simulink library "casper_library"  (Simulink 6.2)
PostLoadFcn:
  | % Stub definitions for mask variables
  | delay_depth=16;
  | n_bits=8;
  | bin_pt=7;
values from neighbouring files (symbols this model uses):
  add_latency = get_var('add_latency', 'defaults', defaults, varargin{:})    [biplex_core_init.m]    (also in butterfly_direct_init.m; dec_fir_init.m = get_var('add_latency','defaults', defaults, varargin{:}); fft_biplex_real_4x_init.m; fft_direct_init.m)
  BitWidth = get_var('BitWidth', 'defaults', defaults, varargin{:})    [biplex_core_init.m]    (also in butterfly_direct_init.m; fft_biplex_init.m; fft_biplex_real_2x_init.m; fft_biplex_real_4x_init.m)
  blockCountBits = ceil(log2(numBlocks))    [address_gen_vacc_v2_mask.m]
  blockRowBits = 0    [address_gen_vacc_v2_mask.m]
  mult_latency = get_var('mult_latency', 'defaults', defaults, varargin{:})    [biplex_core_init.m]    (also in butterfly_direct_init.m; dec_fir_init.m = get_var('mult_latency','defaults', defaults, varargin{:}); fft_biplex_real_4x_init.m; fft_direct_init.m)
  n_inputs = get_var('n_inputs', 'defaults', defaults, varargin{:})    [adder_tree_init.m]    (also in barrel_switcher_init.m; dec_fir_init.m = get_var('n_inputs','defaults', defaults, varargin{:}); fft_init.m; fft_unscrambler_init.m)
undefined symbols (not defined in the file or in its folder): acc_len, ant_bits, bit_growth, bit_rev, BitWidthIn, cmult_4bit_br, cmult_4bit_em, cmult_4bit_sl, CoeffBitWidth, DelayLen, n_ants, n_bits_out, pfb_coeff_gen_calc, PFBSize
libraries: xbsIndex_r3 x2630, casper_library x215, xps_library x24, fft_library x4
(part 4 of 21)

== system casper_library/Downconverter/fir_dbl_col ==
  real1 : Inport  Port=1  LatchInput=off
  imag1 : Inport  Port=2  LatchInput=off
  real2 : Inport  Port=3  LatchInput=off
  imag2 : Inport  Port=4  LatchInput=off
  real_back1 : Inport  Port=5  LatchInput=off
  imag_back1 : Inport  Port=6  LatchInput=off
  real_back2 : Inport  Port=7  LatchInput=off
  imag_back2 : Inport  Port=8  LatchInput=off
  adder_tree1 : Subsystem  AncestorBlock=casper_library/Misc/adder_tree  mask(adder_tree){n_inputs=2, latency=2}
      mask prompts: n_inputs "Number of Inputs"; latency "Add Latency"
      mask help: Sums all inputs using a tree of adds and delays.
      mask init:
      | adder_tree_init(gcb, ...
      |     'n_inputs', n_inputs, ...
      |     'latency', latency);
      settings: AttributesFormatString=latency 2
      mask Help: eval('xlWeb([getenv(''MLIB_ROOT''), ''\doc\html\sp_adder_tree\sp_adder_tree.html''])')
  adder_tree2 : Subsystem  AncestorBlock=casper_library/Misc/adder_tree  mask(adder_tree){n_inputs=2, latency=2}
      mask prompts: n_inputs "Number of Inputs"; latency "Add Latency"
      mask help: Sums all inputs using a tree of adds and delays.
      mask init:
      | adder_tree_init(gcb, ...
      |     'n_inputs', n_inputs, ...
      |     'latency', latency);
      settings: AttributesFormatString=latency 2
      mask Help: eval('xlWeb([getenv(''MLIB_ROOT''), ''\doc\html\sp_adder_tree\sp_adder_tree.html''])')
  c1 : xbsIndex_r3/Constant  const=1  equ=P=C  arith_type=Unsigned  n_bits=1  bin_pt=0  opselect=C  inp2=PCIN>>17  opr=+  inp1=P  carry=CIN  iostate=0  explicit_period=on  period=1  dbl_ovrd=off
  c2 : xbsIndex_r3/Constant  const=1  equ=P=C  arith_type=Unsigned  n_bits=1  bin_pt=0  opselect=C  inp2=PCIN>>17  opr=+  inp1=P  carry=CIN  iostate=0  explicit_period=on  period=1  dbl_ovrd=off
  fir_dbl_tap1 : Subsystem  AncestorBlock=casper_library/Downconverter/fir_dbl_tap  mask(fir_dbl_tap){factor=0.1, add_latency=2, mult_latency=3}
      mask prompts: add_latency "Add latency"; mult_latency "Mult latency"
  fir_dbl_tap2 : Subsystem  AncestorBlock=casper_library/Downconverter/fir_dbl_tap  mask(fir_dbl_tap){factor=0.2, add_latency=2, mult_latency=3}
      mask prompts: add_latency "Add latency"; mult_latency "Mult latency"
  real_out1 : Outport
  imag_out1 : Outport  Port=2
  real_out2 : Outport  Port=3
  imag_out2 : Outport  Port=4
  real_back_out1 : Outport  Port=5
  imag_back_out1 : Outport  Port=6
  real_back_out2 : Outport  Port=7
  imag_back_out2 : Outport  Port=8
  real_sum : Outport  Port=9
  imag_sum : Outport  Port=10
  wires:
  c1/1 -> adder_tree1/1(sync)
  c2/1 -> adder_tree2/1(sync)
  adder_tree1/2(dout) -> real_sum/1
  adder_tree2/2(dout) -> imag_sum/1
  real1/1 -> fir_dbl_tap1/1(a)
  imag1/1 -> fir_dbl_tap1/2(b)
  real_back2/1 -> fir_dbl_tap1/3(c)
  imag_back2/1 -> fir_dbl_tap1/4(d)
  fir_dbl_tap1/1(a_out) -> real_out1/1
  fir_dbl_tap1/2(b_out) -> imag_out1/1
  fir_dbl_tap1/3(c_out) -> real_back_out2/1
  fir_dbl_tap1/4(d_out) -> imag_back_out2/1
  fir_dbl_tap1/5(real) -> adder_tree1/2(din1)
  fir_dbl_tap1/6(imag) -> adder_tree2/2(din1)
  real2/1 -> fir_dbl_tap2/1(a)
  imag2/1 -> fir_dbl_tap2/2(b)
  real_back1/1 -> fir_dbl_tap2/3(c)
  imag_back1/1 -> fir_dbl_tap2/4(d)
  fir_dbl_tap2/1(a_out) -> real_out2/1
  fir_dbl_tap2/2(b_out) -> imag_out2/1
  fir_dbl_tap2/3(c_out) -> real_back_out1/1
  fir_dbl_tap2/4(d_out) -> imag_back_out1/1
  fir_dbl_tap2/5(real) -> adder_tree1/3(din2)
  fir_dbl_tap2/6(imag) -> adder_tree2/3(din2)

== system casper_library/Downconverter/fir_dbl_tap ==
  a : Inport  Port=1  LatchInput=off
  b : Inport  Port=2  LatchInput=off
  c : Inport  Port=3  LatchInput=off
  d : Inport  Port=4  LatchInput=off
  AddSub : xbsIndex_r3/AddSub  mode=Addition  precision=User Defined  arith_type="Signed  (2's comp)"  n_bits=18  bin_pt=16  quantization=Truncate  overflow=Wrap  latency=add_latency  explicit_period=on  period=1  use_carryin=off  use_carryout=off  en=off  dbl_ovrd=off  show_param=off  use_core=on  pipeline=off  use_rpm=on  gen_core=off
      settings: xl_area=[0, 0, 0, 0, 0, 0, 0]
  AddSub1 : xbsIndex_r3/AddSub  mode=Addition  precision=User Defined  arith_type="Signed  (2's comp)"  n_bits=18  bin_pt=16  quantization=Truncate  overflow=Wrap  latency=add_latency  explicit_period=on  period=1  use_carryin=off  use_carryout=off  en=off  dbl_ovrd=off  show_param=off  use_core=on  pipeline=off  use_rpm=on  gen_core=off
      settings: xl_area=[0, 0, 0, 0, 0, 0, 0]
  Constant : xbsIndex_r3/Constant  const=factor  equ=P=C  arith_type="Signed  (2's comp)"  n_bits=18  bin_pt=17  opselect=C  inp2=PCIN>>17  opr=+  inp1=P  carry=CIN  iostate=0  explicit_period=on  period=1  dbl_ovrd=off
  Mult : xbsIndex_r3/Mult  precision=Full  arith_type="Signed  (2's comp)"  n_bits=18  bin_pt=17  quantization=Truncate  overflow=Wrap  latency=mult_latency  explicit_period=off  period=1  en=off  dbl_ovrd=off  show_param=on  mult_type=Parallel  oversample=2  use_embedded=on  pipeline=on  use_rpm=off  placement_style=Rectangular Shape  gen_core=off
      settings: xl_area=[0, 0, 0, 0, 0, 0, 0]
  Mult1 : xbsIndex_r3/Mult  precision=Full  arith_type="Signed  (2's comp)"  n_bits=18  bin_pt=17  quantization=Truncate  overflow=Wrap  latency=mult_latency  explicit_period=off  period=1  en=off  dbl_ovrd=off  show_param=on  mult_type=Parallel  oversample=2  use_embedded=on  pipeline=on  use_rpm=off  placement_style=Rectangular Shape  gen_core=off
      settings: xl_area=[0, 0, 0, 0, 0, 0, 0]
  Register{,1..3} (4 alike) : xbsIndex_r3/Register  init=0  reg_only_valid=off  explicit_period=on  period=1  rst=off  en=off  out_en=off  dbl_ovrd=off  show_param=off
      settings: xl_area=[0, 0, 0, 0, 0, 0, 0]
  a_out : Outport
  b_out : Outport  Port=2
  c_out : Outport  Port=3
  d_out : Outport  Port=4
  real : Outport  Port=5
  imag : Outport  Port=6
  wires:
  AddSub1/1 -> Mult/2
  AddSub/1 -> Mult1/2
  d/1 -> AddSub1/2, Register3/1
  c/1 -> AddSub/2, Register2/1
  b/1 -> AddSub1/1, Register1/1
  a/1 -> AddSub/1, Register/1
  Register2/1 -> c_out/1
  Register3/1 -> d_out/1
  Mult1/1 -> real/1
  Mult/1 -> imag/1
  Constant/1 -> Mult1/1, Mult/1
  Register/1 -> a_out/1
  Register1/1 -> b_out/1

== system casper_library/Downconverter/fir_tap ==
  a : Inport  Port=1  LatchInput=off
  b : Inport  Port=2  LatchInput=off
  Constant : xbsIndex_r3/Constant  const=factor  equ=P=C  arith_type="Signed  (2's comp)"  n_bits=18  bin_pt=17  opselect=C  inp2=PCIN>>17  opr=+  inp1=P  carry=CIN  iostate=0  explicit_period=on  period=1  dbl_ovrd=off
  Mult : xbsIndex_r3/Mult  precision=Full  arith_type="Signed  (2's comp)"  n_bits=18  bin_pt=17  quantization=Truncate  overflow=Wrap  latency=latency  explicit_period=on  period=1  en=off  dbl_ovrd=off  show_param=on  mult_type=Parallel  oversample=2  use_embedded=on  pipeline=on  use_rpm=off  placement_style=Rectangular Shape  gen_core=off
      settings: xl_area=[0, 0, 0, 0, 0, 0, 0]
  Mult1 : xbsIndex_r3/Mult  precision=Full  arith_type="Signed  (2's comp)"  n_bits=18  bin_pt=17  quantization=Truncate  overflow=Wrap  latency=latency  explicit_period=on  period=1  en=off  dbl_ovrd=off  show_param=on  mult_type=Parallel  oversample=2  use_embedded=on  pipeline=on  use_rpm=off  placement_style=Rectangular Shape  gen_core=off
      settings: xl_area=[0, 0, 0, 0, 0, 0, 0]
  Register : xbsIndex_r3/Register  init=0  reg_only_valid=off  explicit_period=on  period=1  rst=off  en=off  out_en=off  dbl_ovrd=off  show_param=off
      settings: xl_area=[0, 0, 0, 0, 0, 0, 0]
  Register1 : xbsIndex_r3/Register  init=0  reg_only_valid=off  explicit_period=on  period=1  rst=off  en=off  out_en=off  dbl_ovrd=off  show_param=off
      settings: xl_area=[0, 0, 0, 0, 0, 0, 0]
  a_out : Outport
  b_out : Outport  Port=2
  real : Outport  Port=3
  imag : Outport  Port=4
  wires:
  Register1/1 -> b_out/1
  Register/1 -> a_out/1
  Constant/1 -> Mult/1, Mult1/1
  a/1 -> Register/1, Mult1/2
  Mult/1 -> imag/1
  b/1 -> Register1/1, Mult/2
  Mult1/1 -> real/1

== system casper_library/Downconverter/lo_const ==
  const : xbsIndex_r3/Constant  const=real(exp(phase*1j))  equ=P=C  arith_type="Signed  (2's comp)"  n_bits=n_bits  bin_pt=n_bits - 1  opselect=C  inp2=PCIN>>17  opr=+  inp1=P  carry=CIN  iostate=0  explicit_period=on  period=1  dbl_ovrd=off
  const1 : xbsIndex_r3/Constant  const=-imag(exp(phase*1j))  equ=P=C  arith_type="Signed  (2's comp)"  n_bits=n_bits  bin_pt=n_bits - 1  opselect=C  inp2=PCIN>>17  opr=+  inp1=P  carry=CIN  iostate=0  explicit_period=on  period=1  dbl_ovrd=off
  sin : Outport
  cos : Outport  Port=2
  wires:
  const/1 -> cos/1
  const1/1 -> sin/1

== system casper_library/Downconverter/lo_osc ==
  sync : Inport  Port=1  LatchInput=off
  SineCosine : xbsIndex_r3/SineCosine  mode=Sine and Cosine  neg_sin=on  neg_cos=off  n_bits=n_bits  latency=latency  sym_output=off  explicit_period=off  period=1  en=off  dbl_ovrd=off  show_param=off  mem_type=Block RAM  pipeline=on  use_rpm=on  gen_core=off
      settings: xl_area=[0, 0, 0, 0, 0, 0, 0]
  counter : xbsIndex_r3/Counter  cnt_type=Free Running  n_bits=counter_width  bin_pt=0  arith_type=Unsigned  start_count=counter_start  cnt_to=Inf  cnt_by_val=counter_step  operation=Up  explicit_period=off  period=1  load_pin=off  rst=on  en=off  dbl_ovrd=off  show_param=off  use_rpm=on  gen_core=off
      settings: xl_area=[0, 0, 0, 0, 0, 0, 0]
  sin : Outport
  cos : Outport  Port=2
  wires:
  counter/1 -> SineCosine/1
  SineCosine/2 -> cos/1
  SineCosine/1 -> sin/1
  sync/1 -> counter/1

== system casper_library/Downconverter/mixer ==
  sync : Inport  Port=1  LatchInput=off
  din1 : Inport  Port=2  LatchInput=off
  din2 : Inport  Port=3  LatchInput=off
  din3 : Inport  Port=4  LatchInput=off
  din4 : Inport  Port=5  LatchInput=off
  dds : Subsystem  AncestorBlock=casper_library/Downconverter/dds  mask(dds){freq_div=16, freq=1, num_lo=4, n_bits=8, latency=2}
      mask prompts: freq_div "Frequency divisions (M)"; freq "Frequency (? / M*2pi)"; num_lo "Parallel LOs"; n_bits "Bit Width"
      mask init:
      | dds_init(gcb, ...
      |     'freq_div', freq_div, ...
      |     'freq', freq, ...
      |     'num_lo', num_lo, ...
      |     'n_bits', n_bits, ...
      |     'latency', latency);
      settings: AttributesFormatString=lo at -1/16
  delay : xbsIndex_r3/Delay  latency=3  reg_retiming=off  explicit_period=off  period=1  en=off  accept_only_valid=off  init_zero=on  dbl_ovrd=off  show_param=off
      settings: xl_area=[0, 0, 0, 0, 0, 0, 0]
  rcmult1 : Subsystem  AncestorBlock=casper_library/Downconverter/rcmult  mask(rcmult){latency=3}
  rcmult2 : Subsystem  AncestorBlock=casper_library/Downconverter/rcmult  mask(rcmult){latency=3}
  rcmult3 : Subsystem  AncestorBlock=casper_library/Downconverter/rcmult  mask(rcmult){latency=3}
  rcmult4 : Subsystem  AncestorBlock=casper_library/Downconverter/rcmult  mask(rcmult){latency=3}
  sync_out : Outport
  real1 : Outport  Port=2
  imag1 : Outport  Port=3
  real2 : Outport  Port=4
  imag2 : Outport  Port=5
  real3 : Outport  Port=6
  imag3 : Outport  Port=7
  real4 : Outport  Port=8
  imag4 : Outport  Port=9
  wires:
  sync/1 -> delay/1
  delay/1 -> sync_out/1
  din1/1 -> rcmult1/1(d)
  dds/1(sin0) -> rcmult1/2(sin)
  dds/2(cos0) -> rcmult1/3(cos)
  rcmult1/1(real) -> real1/1
  rcmult1/2(imag) -> imag1/1
  din2/1 -> rcmult2/1(d)
  dds/3(sin1) -> rcmult2/2(sin)
  dds/4(cos1) -> rcmult2/3(cos)
  rcmult2/1(real) -> real2/1
  rcmult2/2(imag) -> imag2/1
  din3/1 -> rcmult3/1(d)
  dds/5(sin2) -> rcmult3/2(sin)
  dds/6(cos2) -> rcmult3/3(cos)
  rcmult3/1(real) -> real3/1
  rcmult3/2(imag) -> imag3/1
  din4/1 -> rcmult4/1(d)
  dds/7(sin3) -> rcmult4/2(sin)
  dds/8(cos3) -> rcmult4/3(cos)
  rcmult4/1(real) -> real4/1
  rcmult4/2(imag) -> imag4/1

== system casper_library/Downconverter/rcmult ==
  d : Inport  Port=1  LatchInput=off
  sin : Inport  Port=2  LatchInput=off
  cos : Inport  Port=3  LatchInput=off
  Mult : xbsIndex_r3/Mult  precision=Full  arith_type="Signed  (2's comp)"  n_bits=BitWidth  bin_pt=BitWidth-1  quantization=Truncate  overflow=Wrap  latency=latency  explicit_period=off  period=1  en=off  dbl_ovrd=off  show_param=on  mult_type=Parallel  oversample=2  use_embedded=on  pipeline=on  use_rpm=off  placement_style=Rectangular Shape  gen_core=off
      settings: xl_area=[0, 0, 0, 0, 0, 0, 0]
  Mult1 : xbsIndex_r3/Mult  precision=Full  arith_type="Signed  (2's comp)"  n_bits=BitWidth  bin_pt=BitWidth-1  quantization=Truncate  overflow=Wrap  latency=latency  explicit_period=off  period=1  en=off  dbl_ovrd=off  show_param=on  mult_type=Parallel  oversample=2  use_embedded=on  pipeline=on  use_rpm=off  placement_style=Rectangular Shape  gen_core=off
      settings: xl_area=[0, 0, 0, 0, 0, 0, 0]
  real : Outport
  imag : Outport  Port=2
  wires:
  Mult1/1 -> imag/1
  Mult/1 -> real/1
  d/1 -> Mult1/1, Mult/1
  sin/1 -> Mult1/2
  cos/1 -> Mult/2

== system casper_library/FFTs/Twiddle ==
  coeff_gen : Subsystem
  twiddle : Subsystem  BlockChoice=twiddle_coeff_0
      settings: TemplateBlock=self  MemberBlocks=twiddle_coeff_0,twiddle_coeff_1,twiddle_general_3mult,twiddle_general_4mult,twiddle_stage_2
  twiddle_coeff_0 : Subsystem  mask{BitWidth=18, add_latency=3, mult_latency=4, bram_latency=4}
      mask prompts: BitWidth "Bit Width"; add_latency "Add Latency"; mult_latency "Mult Latency"; bram_latency "BRAM Latency"
      mask init:
      | disp(gcb);
  twiddle_coeff_1 : Subsystem  mask{BitWidth=18, add_latency=3, mult_latency=4, bram_latency=4}
      mask prompts: BitWidth "Bit Width"; add_latency "Add Latency"; mult_latency "Mult Latency"; bram_latency "BRAM Latency"
  twiddle_general_3mult : Subsystem  mask{Coeffs=[0], StepPeriod=0, BitWidth=18, add_latency=3, mult_latency=4, bram_latency=4}
      mask prompts: Coeffs "Coefficients:"; StepPeriod "Coefficient Step Period (2^?)"; BitWidth "Bit Width"; add_latency "Add Latency"; mult_latency "Mult Latency"; bram_latency "BRAM Latency"
  twiddle_general_4mult : Subsystem  mask{Coeffs=[0], StepPeriod=0, BitWidth=18, add_latency=3, mult_latency=4, bram_latency=4}
      mask prompts: Coeffs "Coefficients:"; StepPeriod "Coefficient Step Period (2^?)"; BitWidth "Bit Width"; add_latency "Add Latency"; mult_latency "Mult Latency"; bram_latency "BRAM Latency"
  twiddle_stage_2 : Subsystem  mask{FFTSize=5, BitWidth=18, add_latency=3, mult_latency=4, bram_latency=4}
      mask prompts: FFTSize "Size of FFT: (2^?)"; BitWidth "Bit Width"; add_latency "Add Latency"; mult_latency "Mult Latency"; bram_latency "BRAM Latency"

== system casper_library/FFTs/biplex_core ==
  pol1 : Inport  Port=1  LatchInput=off
  pol2 : Inport  Port=2  LatchInput=off
  sync : Inport  Port=3  LatchInput=off
  shift : Inport  Port=4  LatchInput=off
  fft_stage_1 : Subsystem  mask(fft_stage_n){FFTSize=3, FFTStage=1, BitWidth=18, use_bram=0, CoeffBram=0, MaxCoeffNum=16, quantization=Truncate, overflow=Wrap, add_latency=2, mult_latency=3, bram_latency=2}
      mask prompts: FFTSize "Size of FFT: (2^? pnts)"; FFTStage "Stage of FFT:"; BitWidth "Output Bitwidth:"; use_bram "Implement Delays in BRAM:"; CoeffBram "Store Coefficients in BRAM:"; MaxCoeffNum "Maximum Coefficient Depth: (2^?)"; quantization "Quantization Behavior"; overflow "Overflow Behavior"; add_latency "Add Latency"; mult_latency "Mult Latency"; bram_latency "BRAM Latency"
      mask init: same as casper_library/FFTs/fft_stage_n
      settings: AttributesFormatString=FFTSize=3, FFTStage=1, BitWidth=18
      mask StyleString: edit,edit,edit,edit,edit,edit,popup(Truncate|Round  (unbiased: +/- Inf)|Round  (unbiased: Even Values)),popup(Wrap|Saturate|Error),edit,edit,edit
  fft_stage_2 : casper_library/FFTs/fft_stage_n  FFTSize=3  FFTStage=2  BitWidth=18  use_bram=0  CoeffBram=0  MaxCoeffNum=16  quantization=Truncate  overflow=Wrap  add_latency=2  mult_latency=3  bram_latency=2
      settings: AttributesFormatString=FFTSize=3, FFTStage=2, BitWidth=18
  fft_stage_3 : casper_library/FFTs/fft_stage_n  FFTSize=3  FFTStage=3  BitWidth=18  use_bram=0  CoeffBram=0  MaxCoeffNum=16  quantization=Truncate  overflow=Wrap  add_latency=2  mult_latency=3  bram_latency=2
      settings: AttributesFormatString=FFTSize=3, FFTStage=3, BitWidth=18
  out1 : Outport
  out2 : Outport  Port=2
  of : Outport  Port=3
  sync_out : Outport  Port=4
  wires:
  fft_stage_1/1(out1) -> fft_stage_2/1
  fft_stage_1/2(out2) -> fft_stage_2/2
  fft_stage_1/3(of) -> fft_stage_2/3
  fft_stage_1/4(sync_out) -> fft_stage_2/4
  shift/1 -> fft_stage_2/5, fft_stage_3/5, fft_stage_1/4(shift)
  fft_stage_2/1 -> fft_stage_3/1
  fft_stage_2/2 -> fft_stage_3/2
  fft_stage_2/3 -> fft_stage_3/3
  fft_stage_2/4 -> fft_stage_3/4
  pol1/1 -> fft_stage_1/1(in1)
  pol2/1 -> fft_stage_1/2(in2)
  sync/1 -> fft_stage_1/3(sync)
  fft_stage_3/1 -> out1/1
  fft_stage_3/2 -> out2/1
  fft_stage_3/3 -> of/1
  fft_stage_3/4 -> sync_out/1

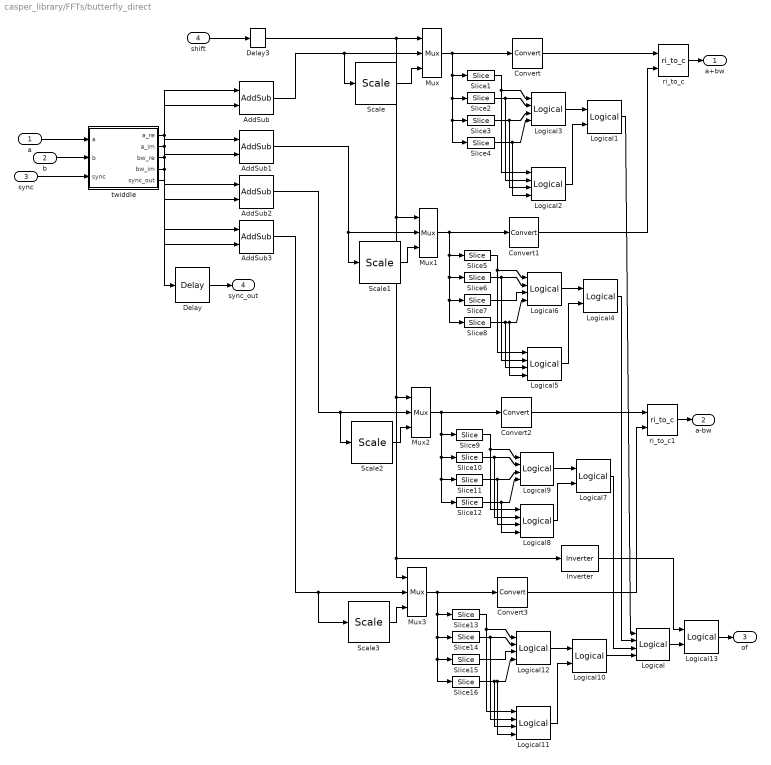
== system casper_library/FFTs/butterfly_direct ==
  a : Inport  Port=1  LatchInput=off
  b : Inport  Port=2  LatchInput=off
  sync : Inport  Port=3  LatchInput=off
  shift : Inport  Port=4  LatchInput=off
  AddSub : xbsIndex_r3/AddSub  mode=Addition  precision=Full  arith_type=Unsigned  n_bits=8  bin_pt=2  quantization=Truncate  overflow=Wrap  latency=add_latency  explicit_period=off  period=1  use_carryin=off  use_carryout=off  en=off  dbl_ovrd=off  show_param=on  use_core=on  pipeline=on  use_rpm=on  gen_core=on
      settings: xl_area=[0, 0, 0, 0, 0, 0, 0]
  AddSub1 : xbsIndex_r3/AddSub  mode=Addition  precision=Full  arith_type=Unsigned  n_bits=8  bin_pt=2  quantization=Truncate  overflow=Wrap  latency=add_latency  explicit_period=off  period=1  use_carryin=off  use_carryout=off  en=off  dbl_ovrd=off  show_param=on  use_core=on  pipeline=on  use_rpm=on  gen_core=on
      settings: xl_area=[0, 0, 0, 0, 0, 0, 0]
  AddSub2 : xbsIndex_r3/AddSub  mode=Subtraction  precision=Full  arith_type=Unsigned  n_bits=8  bin_pt=2  quantization=Truncate  overflow=Wrap  latency=add_latency  explicit_period=off  period=1  use_carryin=off  use_carryout=off  en=off  dbl_ovrd=off  show_param=on  use_core=on  pipeline=on  use_rpm=on  gen_core=on
      settings: xl_area=[0, 0, 0, 0, 0, 0, 0]
  AddSub3 : xbsIndex_r3/AddSub  mode=Subtraction  precision=Full  arith_type=Unsigned  n_bits=8  bin_pt=2  quantization=Truncate  overflow=Wrap  latency=add_latency  explicit_period=off  period=1  use_carryin=off  use_carryout=off  en=off  dbl_ovrd=off  show_param=on  use_core=on  pipeline=on  use_rpm=on  gen_core=on
      settings: xl_area=[0, 0, 0, 0, 0, 0, 0]
  Convert{,1..3} (4 alike) : xbsIndex_r3/Convert  arith_type="Signed  (2's comp)"  n_bits=BitWidth  bin_pt=BitWidth-1  quantization=Truncate  overflow=Wrap  latency=add_latency  explicit_period=off  period=1  dbl_ovrd=off  show_param=off  inserted_by_tool=off  pipeline=off
      settings: xl_area=[0, 0, 0, 0, 0, 0, 0]
  Delay : xbsIndex_r3/Delay  latency=2 * add_latency + 1  reg_retiming=off  explicit_period=off  period=1  en=off  accept_only_valid=off  init_zero=on  dbl_ovrd=off  show_param=off
      settings: xl_area=[0, 0, 0, 0, 0, 0, 0]
  Delay3 : xbsIndex_r3/Delay  latency=1  reg_retiming=off  explicit_period=off  period=1  en=off  accept_only_valid=off  init_zero=on  dbl_ovrd=off  show_param=off
      settings: xl_area=[0, 0, 0, 0, 0, 0, 0]
  Inverter : xbsIndex_r3/Inverter  latency=0  explicit_period=off  period=1  en=off  dbl_ovrd=off  show_param=off
      settings: xl_area=[0, 0, 0, 0, 0, 0, 0]
  Logical : xbsIndex_r3/Logical  logical_function=OR  inputs=4  precision=Full  arith_type=Unsigned  n_bits=8  bin_pt=2  align_bp=on  latency=1  explicit_period=off  period=1  en=off  dbl_ovrd=off  show_param=off
      settings: xl_area=[0, 0, 0, 0, 0, 0, 0]
  Logical{1,4,7,10} (4 alike) : xbsIndex_r3/Logical  logical_function=OR  inputs=2  precision=Full  arith_type=Unsigned  n_bits=8  bin_pt=2  align_bp=off  latency=1  explicit_period=off  period=1  en=off  dbl_ovrd=off  show_param=off
      settings: xl_area=[0, 0, 0, 0, 0, 0, 0]
  Logical{2,5,8,11} (4 alike) : xbsIndex_r3/Logical  logical_function=NOR  inputs=4  precision=Full  arith_type=Unsigned  n_bits=8  bin_pt=2  align_bp=off  latency=1  explicit_period=off  period=1  en=off  dbl_ovrd=off  show_param=off
      settings: xl_area=[0, 0, 0, 0, 0, 0, 0]
  Logical{3,6,9,12} (4 alike) : xbsIndex_r3/Logical  logical_function=AND  inputs=4  precision=Full  arith_type=Unsigned  n_bits=8  bin_pt=2  align_bp=off  latency=1  explicit_period=off  period=1  en=off  dbl_ovrd=off  show_param=off
      settings: xl_area=[0, 0, 0, 0, 0, 0, 0]
  Logical13 : xbsIndex_r3/Logical  logical_function=AND  inputs=2  precision=Full  arith_type=Unsigned  n_bits=8  bin_pt=2  align_bp=off  latency=1  explicit_period=off  period=1  en=off  dbl_ovrd=off  show_param=off
      settings: xl_area=[0, 0, 0, 0, 0, 0, 0]
  Mux{,1..3} (4 alike) : xbsIndex_r3/Mux  inputs=2  precision=Full  arith_type="Signed  (2's comp)"  n_bits=8  bin_pt=2  quantization=Truncate  overflow=Wrap  latency=1  explicit_period=off  period=1  en=off  dbl_ovrd=off  show_param=off  mux_type=off  use_rpm=off  gen_core=off
      settings: xl_area=[0, 0, 0, 0, 0, 0, 0]
  Scale{,1..3} (4 alike) : xbsIndex_r3/Scale  scale_factor=-1  explicit_period=off  period=1  dbl_ovrd=off
  Slice{1,5,9,13} (4 alike) : xbsIndex_r3/Slice  mode=Upper Bit Location + Width  nbits=1  bit1=0  base1=MSB of Input  bit0=0  base0=LSB of Input  boolean_output=on  explicit_period=off  period=1  dbl_ovrd=off
  Slice{2,6,10,14} (4 alike) : xbsIndex_r3/Slice  mode=Upper Bit Location + Width  nbits=1  bit1=-1  base1=MSB of Input  bit0=0  base0=LSB of Input  boolean_output=on  explicit_period=off  period=1  dbl_ovrd=off
  Slice{3,7,11,15} (4 alike) : xbsIndex_r3/Slice  mode=Upper Bit Location + Width  nbits=1  bit1=-2  base1=MSB of Input  bit0=0  base0=LSB of Input  boolean_output=on  explicit_period=off  period=1  dbl_ovrd=off
  Slice{4,8,12,16} (4 alike) : xbsIndex_r3/Slice  mode=Upper Bit Location + Width  nbits=1  bit1=-3  base1=MSB of Input  bit0=0  base0=LSB of Input  boolean_output=on  explicit_period=off  period=1  dbl_ovrd=off
  ri_to_c : casper_library/Misc/ri_to_c
  ri_to_c1 : casper_library/Misc/ri_to_c
  twiddle : Subsystem  BlockChoice=twiddle_general_3mult
      link override twiddle_general_3mult: Coeffs=[exp(-2*pi*1j*(bit_rev(Coeffs, FFTSize-1))/2^FFTSize)]  StepPeriod=4  BitWidth=18  add_latency=4  mult_latency=5  bram_latency=6
      link override twiddle_general_3mult/coeff_gen: BlockChoice=br_coeff_gen
      link override twiddle_general_3mult/coeff_gen/br_coeff_gen: Coeffs=[1 2 3 4 5 6 7]  StepPeriod=4  BitWidth=10  bram_latency=6
      link override twiddle_general_3mult/coeff_gen/br_coeff_gen/ROM: distributed_mem=off
      link override twiddle_general_3mult/coeff_gen/br_coeff_gen/ROM1: distributed_mem=off
      settings: AttributesFormatString=%<BlockChoice>  TemplateBlock=casper_library/FFTs/Twiddle/twiddle  MemberBlocks=twiddle_coeff_0,twiddle_coeff_1,twiddle_general_3mult,twiddle_general_4mult,twiddle_stage_2
  a+bw : Outport
  a-bw : Outport  Port=2
  of : Outport  Port=3
  sync_out : Outport  Port=4
  wires:
  twiddle/5(sync_out) -> Delay/1
  twiddle/4(bw_im) -> AddSub3/2, AddSub1/2
  twiddle/3(bw_re) -> AddSub2/2, AddSub/2
  twiddle/2(a_im) -> AddSub3/1, AddSub1/1
  twiddle/1(a_re) -> AddSub2/1, AddSub/1
  sync/1 -> twiddle/3(sync)
  b/1 -> twiddle/2(b)
  a/1 -> twiddle/1(a)
  ri_to_c/1 -> a+bw/1
  ri_to_c1/1 -> a-bw/1
  Delay/1 -> sync_out/1
  AddSub/1 -> Mux/2, Scale/1
  AddSub1/1 -> Mux1/2, Scale1/1
  shift/1 -> Delay3/1
  Mux/1 -> Convert/1, Slice1/1, Slice2/1, Slice3/1, Slice4/1
  Scale/1 -> Mux/3
  Convert/1 -> ri_to_c/1
  Slice1/1 -> Logical3/1, Logical2/1
  Slice2/1 -> Logical3/2, Logical2/2
  Slice3/1 -> Logical3/3, Logical2/3
  Slice4/1 -> Logical3/4, Logical2/4
  Logical3/1 -> Logical1/1
  Logical2/1 -> Logical1/2
  Logical1/1 -> Logical/1
  Mux1/1 -> Convert1/1, Slice5/1, Slice6/1, Slice7/1, Slice8/1
  Scale1/1 -> Mux1/3
  Convert1/1 -> ri_to_c/2
  Slice5/1 -> Logical6/1, Logical5/1
  Slice6/1 -> Logical6/2, Logical5/2
  Slice7/1 -> Logical6/3
  Slice8/1 -> Logical6/4, Logical5/4, Logical5/3
  Logical6/1 -> Logical4/1
  Logical5/1 -> Logical4/2
  Logical4/1 -> Logical/2
  Mux2/1 -> Convert2/1, Slice9/1, Slice10/1, Slice11/1, Slice12/1
  Scale2/1 -> Mux2/3
  Convert2/1 -> ri_to_c1/1
  Slice9/1 -> Logical9/1, Logical8/1
  Slice10/1 -> Logical9/2, Logical8/2
  Slice11/1 -> Logical9/3, Logical8/3
  Slice12/1 -> Logical9/4, Logical8/4
  Logical9/1 -> Logical7/1
  Logical8/1 -> Logical7/2
  AddSub2/1 -> Mux2/2, Scale2/1
  Mux3/1 -> Convert3/1, Slice13/1, Slice14/1, Slice15/1, Slice16/1
  Scale3/1 -> Mux3/3
  Convert3/1 -> ri_to_c1/2
  Slice13/1 -> Logical12/1, Logical11/1
  Slice14/1 -> Logical12/2, Logical11/2
  Slice15/1 -> Logical12/3
  Slice16/1 -> Logical12/4, Logical11/4, Logical11/3
  Logical12/1 -> Logical10/1
  Logical11/1 -> Logical10/2
  Logical10/1 -> Logical/4
  AddSub3/1 -> Mux3/2, Scale3/1
  Logical7/1 -> Logical/3
  Delay3/1 -> Mux/1, Mux1/1, Mux2/1, Mux3/1, Inverter/1
  Logical/1 -> Logical13/2
  Logical13/1 -> of/1
  Inverter/1 -> Logical13/1

== system casper_library/FFTs/fft ==
  sync : Inport  Port=1  LatchInput=off
  shift : Inport  Port=2  LatchInput=off
  in0 : Inport  Port=3  LatchInput=off
  in1 : Inport  Port=4  LatchInput=off
  in2 : Inport  Port=5  LatchInput=off
  in3 : Inport  Port=6  LatchInput=off
  fft_biplex0 : casper_library/FFTs/fft_biplex  FFTSize=3  BitWidth=18  quantization=Truncate  overflow=Wrap  add_latency=2  mult_latency=3  bram_latency=2
      settings: AttributesFormatString=FFTSize=3, BitWidth=18
  fft_biplex1 : casper_library/FFTs/fft_biplex  FFTSize=3  BitWidth=18  quantization=Truncate  overflow=Wrap  add_latency=2  mult_latency=3  bram_latency=2
      settings: AttributesFormatString=FFTSize=3, BitWidth=18
  fft_direct : casper_library/FFTs/fft_direct  FFTSize=2  BitWidth=18  add_latency=2  mult_latency=3  bram_latency=2  quantization=Truncate  overflow=Wrap  MapTail=1  LargerFFTSize=5  StartStage=4
      settings: AttributesFormatString=FFTSize=2
  fft_unscrambler : casper_library/FFTs/fft_unscrambler  FFTSize=5  n_inputs=2  bram_latency=2
      settings: AttributesFormatString=FFTSize=5, n_inputs=2
  slice : xbsIndex_r3/Slice  mode=Lower Bit Location + Width  nbits=2  bit1=0  base1=MSB of Input  bit0=3  base0=LSB of Input  boolean_output=off  explicit_period=off  period=1  dbl_ovrd=off
  sync_out : Outport
  out0 : Outport  Port=2
  out1 : Outport  Port=3
  out2 : Outport  Port=4
  out3 : Outport  Port=5
  wires:
  in0/1 -> fft_biplex0/1
  in1/1 -> fft_biplex0/2
  shift/1 -> fft_biplex0/4, fft_biplex1/4, slice/1
  sync/1 -> fft_biplex0/3, fft_biplex1/3
  in2/1 -> fft_biplex1/1
  in3/1 -> fft_biplex1/2
  slice/1 -> fft_direct/2
  fft_biplex0/4 -> fft_direct/1
  fft_biplex0/1 -> fft_direct/3
  fft_biplex0/2 -> fft_direct/4
  fft_biplex1/1 -> fft_direct/5
  fft_biplex1/2 -> fft_direct/6
  fft_direct/1 -> fft_unscrambler/1
  fft_unscrambler/1 -> sync_out/1
  fft_direct/2 -> fft_unscrambler/2
  fft_unscrambler/2 -> out0/1
  fft_direct/3 -> fft_unscrambler/3
  fft_unscrambler/3 -> out1/1
  fft_direct/4 -> fft_unscrambler/4
  fft_unscrambler/4 -> out2/1
  fft_direct/5 -> fft_unscrambler/5
  fft_unscrambler/5 -> out3/1

== system casper_library/FFTs/fft_biplex ==
  pol1 : Inport  Port=1  LatchInput=off
  pol2 : Inport  Port=2  LatchInput=off
  sync : Inport  Port=3  LatchInput=off
  shift : Inport  Port=4  LatchInput=off
  biplex_core : casper_library/FFTs/biplex_core  FFTSize=3  BitWidth=18  quantization=Truncate  overflow=Wrap  add_latency=2  mult_latency=3  bram_latency=2
      settings: AttributesFormatString=FFTSize=3
  biplex_cplx_unscrambler : Subsystem  mask{FFTSize=3, bram_latency=2}
      mask prompts: FFTSize "Size of FFT: (2^? pnts)"; bram_latency "BRAM Latency"
      mask init:
      | blk = gcb;
      | map = bit_reverse(0:2^(FFTSize-1)-1, FFTSize-1);
      | set_param([blk,'/reorder'],'map',mat2str([map,map+2^(FFTSize-1)]));
      | set_param([blk,'/reorder'],'bram_latency', num2str(bram_latency));
      | set_param([blk,'/reorder1'],'map',mat2str([map+2^(FFTSize-1),map]));
      | set_param([blk,'/reorder1'],'bram_latency', num2str(bram_latency));
  pol1_out : Outport
  pol2_out : Outport  Port=2
  of : Outport  Port=3
  sync_out : Outport  Port=4
  wires:
  biplex_core/3 -> of/1
  biplex_cplx_unscrambler/1(pol1) -> pol1_out/1
  shift/1 -> biplex_core/4
  sync/1 -> biplex_core/3
  pol2/1 -> biplex_core/2
  pol1/1 -> biplex_core/1
  biplex_core/1 -> biplex_cplx_unscrambler/1(even)
  biplex_core/2 -> biplex_cplx_unscrambler/2(odd)
  biplex_core/4 -> biplex_cplx_unscrambler/3(sync)
  biplex_cplx_unscrambler/2(pol2) -> pol2_out/1
  biplex_cplx_unscrambler/3(sync_out) -> sync_out/1

== system casper_library/FFTs/fft_biplex_real_2x ==
  pol1 : Inport  Port=1  LatchInput=off
  pol2 : Inport  Port=2  LatchInput=off
  pol3 : Inport  Port=3  LatchInput=off
  pol4 : Inport  Port=4  LatchInput=off
  sync : Inport  Port=5  LatchInput=off
  shift : Inport  Port=6  LatchInput=off
  bi_real_unscr_2x : Subsystem  mask{FFTSize=FFTSize, n_bits=BitWidth, add_latency=add_latency, bram_latency=bram_latency}
      mask prompts: FFTSize "Size of FFT (2^?):"; n_bits "Sample Bit Width"; add_latency "Add Latency"; bram_latency "BRAM Latency"
      mask init:
      | blk = gcb;
      | 
      | set_param([blk,'/reorder'],'map', mat2str(bit_reverse(0:2^(FFTSize-1)-1, FFTSize-1)));
      | set_param([blk,'/reorder'],'bram_latency', num2str(bram_latency));
      | set_param([blk,'/reorder1'],'map', mat2str(bit_reverse(2^(FFTSize-1)-1:-1:0, FFTSize-1)));
      | set_param([blk,'/reorder1'],'bram_latency', num2str(bram_latency));
  biplex_core : casper_library/FFTs/biplex_core  FFTSize=4  BitWidth=18  quantization=Truncate  overflow=Saturate  add_latency=2  mult_latency=3  bram_latency=2
      settings: AttributesFormatString=FFTSize=4
  ri_to_c : Subsystem
  ri_to_c1 : Subsystem
  pol12_out : Outport
  pol34_out : Outport  Port=2
  of : Outport  Port=3
  sync_out : Outport  Port=4
  wires:
  bi_real_unscr_2x/3(sync_out) -> sync_out/1
  bi_real_unscr_2x/2(pol34_out) -> pol34_out/1
  bi_real_unscr_2x/1(pol12_out) -> pol12_out/1
  shift/1 -> biplex_core/4
  sync/1 -> biplex_core/3
  pol4/1 -> ri_to_c1/2(im)
  ri_to_c1/1(c) -> biplex_core/2
  pol3/1 -> ri_to_c1/1(re)
  pol2/1 -> ri_to_c/2(im)
  ri_to_c/1(c) -> biplex_core/1
  pol1/1 -> ri_to_c/1(re)
  biplex_core/3 -> of/1
  biplex_core/1 -> bi_real_unscr_2x/1(even)
  biplex_core/2 -> bi_real_unscr_2x/2(odd)
  biplex_core/4 -> bi_real_unscr_2x/3(sync)

== system casper_library/FFTs/fft_biplex_real_4x ==
  pol1 : Inport  Port=1  LatchInput=off
  pol2 : Inport  Port=2  LatchInput=off
  pol3 : Inport  Port=3  LatchInput=off
  pol4 : Inport  Port=4  LatchInput=off
  sync : Inport  Port=5  LatchInput=off
  shift : Inport  Port=6  LatchInput=off
  bi_real_unscr_4x : Subsystem  mask{FFTSize=4, bram_latency=2}
      mask prompts: FFTSize "Size of FFT (2^?):"; bram_latency "BRAM Latency"
      mask init:
      | blk = gcb;
      | 
      | set_param([blk,'/reorder'],'map', mat2str(bit_reverse(0:2^(FFTSize-1)-1, FFTSize-1)));
      | set_param([blk,'/reorder'],'bram_latency', num2str(bram_latency));
      | set_param([blk,'/reorder1'],'map', mat2str(bit_reverse(2^(FFTSize-1)-1:-1:0, FFTSize-1)));
      | set_param([blk,'/reorder1'],'bram_latency', num2str(bram_latency));
      | set_param([blk,'/reorder2'],'map', mat2str(2^(FFTSize-1)-1:-1:0));
      | set_param([blk,'/reorder2'],'bram_latency', num2str(bram_latency));
  biplex_core : casper_library/FFTs/biplex_core  FFTSize=4  BitWidth=18  quantization=Truncate  overflow=Wrap  add_latency=2  mult_latency=3  bram_latency=2
      settings: AttributesFormatString=FFTSize=4
  ri_to_c : Subsystem
  ri_to_c1 : Subsystem
  pol1_out : Outport
  pol2_out : Outport  Port=2
  pol3_out : Outport  Port=3
  pol4_out : Outport  Port=4
  of : Outport  Port=5
  sync_out : Outport  Port=6
  wires:
  bi_real_unscr_4x/5(sync_out) -> sync_out/1
  bi_real_unscr_4x/4(pol4_out) -> pol4_out/1
  bi_real_unscr_4x/3(pol3_out) -> pol3_out/1
  bi_real_unscr_4x/2(pol2_out) -> pol2_out/1
  bi_real_unscr_4x/1(pol1_out) -> pol1_out/1
  shift/1 -> biplex_core/4
  sync/1 -> biplex_core/3
  pol4/1 -> ri_to_c1/2(im)
  ri_to_c1/1(c) -> biplex_core/2
  pol3/1 -> ri_to_c1/1(re)
  pol2/1 -> ri_to_c/2(im)
  ri_to_c/1(c) -> biplex_core/1
  pol1/1 -> ri_to_c/1(re)
  biplex_core/3 -> of/1
  biplex_core/1 -> bi_real_unscr_4x/1(even)
  biplex_core/2 -> bi_real_unscr_4x/2(odd)
  biplex_core/4 -> bi_real_unscr_4x/3(sync)

== system casper_library/FFTs/fft_direct ==
  sync : Inport  Port=1  LatchInput=off
  shift : Inport  Port=2  LatchInput=off
  in0 : Inport  Port=3  LatchInput=off
  in1 : Inport  Port=4  LatchInput=off
  in2 : Inport  Port=5  LatchInput=off
  in3 : Inport  Port=6  LatchInput=off
  butterfly1_0 : casper_library/FFTs/butterfly_direct  FFTSize=5  Coeffs=[ 0 2 1 3 0 2 1 3]  StepPeriod=0  BitWidth=BitWidth  add_latency=add_latency  mult_latency=mult_latency  bram_latency=bram_latency  use_bram=1  quantization=Truncate  overflow=Wrap
      settings: AttributesFormatString=|
      | FFTSize=5, Coeffs=[0  2  1  3  0  2  1  3],
      |  StepPeriod=0, BitWidth=18
  butterfly1_1 : casper_library/FFTs/butterfly_direct  FFTSize=5  Coeffs=[ 0 2 1 3 0 2 1 3]  StepPeriod=0  BitWidth=BitWidth  add_latency=add_latency  mult_latency=mult_latency  bram_latency=bram_latency  use_bram=1  quantization=Truncate  overflow=Wrap
      settings: AttributesFormatString=|
      | FFTSize=5, Coeffs=[0  2  1  3  0  2  1  3],
      |  StepPeriod=0, BitWidth=18
  butterfly2_0 : casper_library/FFTs/butterfly_direct  FFTSize=5  Coeffs=[ 0 4 2 6 1 5 3 7]  StepPeriod=0  BitWidth=BitWidth  add_latency=add_latency  mult_latency=mult_latency  bram_latency=bram_latency  use_bram=1  quantization=Truncate  overflow=Wrap
      settings: AttributesFormatString=|
      | FFTSize=5, Coeffs=[0  4  2  6  1  5  3  7],
      |  StepPeriod=0, BitWidth=18
  butterfly2_1 : casper_library/FFTs/butterfly_direct  FFTSize=5  Coeffs=[ 0 4 2 6 1 5 3 7]  StepPeriod=0  BitWidth=BitWidth  add_latency=add_latency  mult_latency=mult_latency  bram_latency=bram_latency  use_bram=1  quantization=Truncate  overflow=Wrap
      settings: AttributesFormatString=|
      | FFTSize=5, Coeffs=[0  4  2  6  1  5  3  7],
      |  StepPeriod=0, BitWidth=18
  node0_{0..3} (4 alike) : xbsIndex_r3/Delay  latency=0  reg_retiming=off  explicit_period=off  period=1  en=off  accept_only_valid=off  init_zero=on  dbl_ovrd=off  show_param=off
      settings: xl_area=[0, 0, 0, 0, 0, 0, 0]
  node1_{0..3} (4 alike) : xbsIndex_r3/Delay  latency=0  reg_retiming=off  explicit_period=off  period=1  en=off  accept_only_valid=off  init_zero=on  dbl_ovrd=off  show_param=off
      settings: xl_area=[0, 0, 0, 0, 0, 0, 0]
  node2_{0..3} (4 alike) : xbsIndex_r3/Delay  latency=0  reg_retiming=off  explicit_period=off  period=1  en=off  accept_only_valid=off  init_zero=on  dbl_ovrd=off  show_param=off
      settings: xl_area=[0, 0, 0, 0, 0, 0, 0]
  slice0 : xbsIndex_r3/Slice  mode=Lower Bit Location + Width  nbits=1  bit1=0  base1=MSB of Input  bit0=0  base0=LSB of Input  boolean_output=on  explicit_period=off  period=1  dbl_ovrd=off
  slice1 : xbsIndex_r3/Slice  mode=Lower Bit Location + Width  nbits=1  bit1=0  base1=MSB of Input  bit0=1  base0=LSB of Input  boolean_output=on  explicit_period=off  period=1  dbl_ovrd=off
  sync_out : Outport
  out0 : Outport  Port=2
  out1 : Outport  Port=3
  out2 : Outport  Port=4
  out3 : Outport  Port=5
  wires:
  in0/1 -> node0_0/1
  in1/1 -> node0_1/1
  in2/1 -> node0_2/1
  in3/1 -> node0_3/1
  shift/1 -> slice0/1, slice1/1
  node2_0/1 -> out0/1
  node2_1/1 -> out2/1
  node2_2/1 -> out1/1
  node2_3/1 -> out3/1
  node0_0/1 -> butterfly1_0/1
  node0_2/1 -> butterfly1_0/2
  butterfly1_0/1 -> node1_0/1
  butterfly1_0/2 -> node1_2/1
  sync/1 -> butterfly1_0/3, butterfly1_1/3
  slice0/1 -> butterfly1_0/4, butterfly1_1/4
  node0_1/1 -> butterfly1_1/1
  node0_3/1 -> butterfly1_1/2
  butterfly1_1/1 -> node1_1/1
  butterfly1_1/2 -> node1_3/1
  node1_0/1 -> butterfly2_0/1
  node1_1/1 -> butterfly2_0/2
  butterfly2_0/1 -> node2_0/1
  butterfly2_0/2 -> node2_1/1
  butterfly1_0/4 -> butterfly2_0/3
  butterfly2_0/4 -> sync_out/1
  slice1/1 -> butterfly2_0/4, butterfly2_1/4
  node1_2/1 -> butterfly2_1/1
  node1_3/1 -> butterfly2_1/2
  butterfly2_1/1 -> node2_2/1
  butterfly2_1/2 -> node2_3/1
  butterfly1_1/4 -> butterfly2_1/3

== system casper_library/FFTs/fft_stage_n ==
  in1 : Inport  Port=1  LatchInput=off
  in2 : Inport  Port=2  LatchInput=off
  of_in : Inport  Port=3  LatchInput=off
  sync : Inport  Port=4  LatchInput=off
  shift : Inport  Port=5  LatchInput=off
  Counter : xbsIndex_r3/Counter  cnt_type=Free Running  n_bits=FFTSize-FFTStage+1  bin_pt=0  arith_type=Unsigned  start_count=0  cnt_to=Inf  cnt_by_val=1  operation=Up  explicit_period=off  period=1  load_pin=off  rst=on  en=off  dbl_ovrd=off  show_param=off  use_rpm=off  gen_core=on
      settings: xl_area=[0, 0, 0, 0, 0, 0, 0]
  Delay : xbsIndex_r3/Delay  latency=1  reg_retiming=off  explicit_period=off  period=1  en=off  accept_only_valid=off  init_zero=on  dbl_ovrd=off  show_param=off
      settings: xl_area=[0, 0, 0, 0, 0, 0, 0]
  Logical1 : xbsIndex_r3/Logical  logical_function=OR  inputs=2  precision=Full  arith_type=Unsigned  n_bits=8  bin_pt=2  align_bp=on  latency=1  explicit_period=on  period=1  en=off  dbl_ovrd=off  show_param=off
      settings: xl_area=[0, 0, 0, 0, 0, 0, 0]
  Mux : xbsIndex_r3/Mux  inputs=2  precision=Full  arith_type="Signed  (2's comp)"  n_bits=8  bin_pt=2  quantization=Truncate  overflow=Wrap  latency=1  explicit_period=off  period=1  en=off  dbl_ovrd=off  show_param=off  mux_type=off  use_rpm=off  gen_core=on
      settings: xl_area=[0, 0, 0, 0, 0, 0, 0]
  Mux1 : xbsIndex_r3/Mux  inputs=2  precision=Full  arith_type="Signed  (2's comp)"  n_bits=8  bin_pt=2  quantization=Truncate  overflow=Wrap  latency=1  explicit_period=off  period=1  en=off  dbl_ovrd=off  show_param=off  mux_type=off  use_rpm=off  gen_core=on
      settings: xl_area=[0, 0, 0, 0, 0, 0, 0]
  Slice : xbsIndex_r3/Slice  Orientation=up  mode=Lower Bit Location + Width  nbits=1  bit1=-(FFTStage - 1)  base1=MSB of Input  bit0=FFTStage - 1  base0=LSB of Input  boolean_output=on  explicit_period=off  period=1  dbl_ovrd=off
  Slice1 : xbsIndex_r3/Slice  mode=Upper Bit Location + Width  nbits=1  bit1=0  base1=MSB of Input  bit0=0  base0=LSB of Input  boolean_output=off  explicit_period=off  period=1  dbl_ovrd=off
  butterfly_direct : casper_library/FFTs/butterfly_direct  FFTSize=5  Coeffs=[0 1 2 3]  StepPeriod=2  BitWidth=18  add_latency=3  mult_latency=2  bram_latency=2  use_bram=0  quantization=Truncate  overflow=Wrap
      link override twiddle/twiddle_general_3mult/coeff_gen/br_coeff_gen/ROM: distributed_mem=off
      link override twiddle/twiddle_general_3mult/coeff_gen/br_coeff_gen/ROM1: distributed_mem=off
      settings: AttributesFormatString=|
      | FFTSize=5, Coeffs=[0  1  2  3],
      |  StepPeriod=2, BitWidth=18
  delay_b : Subsystem  BlockChoice=delay_slr
      link override delay_bram: bram_latency=bram_latency  DelayLen=2^(FFTSize-FFTStage)
      link override delay_slr: DelayLen=2^(FFTSize-FFTStage)
      settings: AttributesFormatString=%<BlockChoice>  TemplateBlock=casper_library/Delays/delay  MemberBlocks=delay_bram,delay_slr
  delay_f : Subsystem  BlockChoice=delay_slr
      link override delay_bram: bram_latency=bram_latency  DelayLen=2^(FFTSize-FFTStage)
      link override delay_slr: DelayLen=2^(FFTSize-FFTStage)
      settings: AttributesFormatString=%<BlockChoice>  TemplateBlock=casper_library/Delays/delay  MemberBlocks=delay_bram,delay_slr
  sync_delay : casper_library/Delays/sync_delay  DelayLen=2^(FFTSize - FFTStage)
  out1 : Outport
  out2 : Outport  Port=2
  of : Outport  Port=3
  sync_out : Outport  Port=4
  wires:
  shift/1 -> Slice/1
  of_in/1 -> Logical1/2
  Logical1/1 -> of/1
  Delay/1 -> sync_delay/1
  sync/1 -> Counter/1, Delay/1
  Counter/1 -> Slice1/1
  Mux/1 -> butterfly_direct/2
  Mux1/1 -> delay_b/1(In1)
  delay_f/1(Out1) -> Mux1/3, Mux/2
  in1/1 -> Mux/3, Mux1/2
  Slice1/1 -> Mux/1, Mux1/1
  in2/1 -> delay_f/1(In1)
  delay_b/1(Out1) -> butterfly_direct/1
  sync_delay/1 -> butterfly_direct/3
  Slice/1 -> butterfly_direct/4
  butterfly_direct/3 -> Logical1/1
  butterfly_direct/2 -> out2/1
  butterfly_direct/1 -> out1/1
  butterfly_direct/4 -> sync_out/1

== system casper_library/FFTs/fft_unscrambler ==
  sync : Inport  Port=1  LatchInput=off
  In1 : Inport  Port=2  LatchInput=off
  In2 : Inport  Port=3  LatchInput=off
  In3 : Inport  Port=4  LatchInput=off
  In4 : Inport  Port=5  LatchInput=off
  const : xbsIndex_r3/Constant  const=1  equ=P=C  arith_type=Boolean  n_bits=1  bin_pt=0  opselect=C  inp2=PCIN>>17  opr=+  inp1=P  carry=CIN  iostate=0  explicit_period=on  period=1  dbl_ovrd=off
  reorder : Subsystem  AncestorBlock=casper_library/Reorder/reorder  mask(reorder){map=[0 4 1 5 2 6 3 7], n_inputs=4, bram_latency=2, map_latency=1, double_buffer=0}
      mask prompts: map "Output Order:"; n_inputs "Number of inputs"; bram_latency "BRAM Latency"; map_latency "Map Latency"; double_buffer "Double Buffer"
      mask init:
      | reorder_init(gcb, ...
      |     'map', map, ...
      |     'n_inputs', n_inputs, ...
      |     'bram_latency', bram_latency, ...
      |     'map_latency', map_latency, ...
      |     'double_buffer', double_buffer);
      settings: AttributesFormatString=order=3
  square_transposer : Subsystem  AncestorBlock=casper_library/Reorder/square_transposer  mask(square_transposer){n_inputs=2}
      mask prompts: n_inputs "Number of inputs (2^?):"
      mask init:
      | square_transposer_init(gcb,...
      |     'n_inputs', n_inputs);
      settings: AttributesFormatString=n_inputs=2
  sync_out : Outport
  Out1 : Outport  Port=2
  Out2 : Outport  Port=3
  Out3 : Outport  Port=4
  Out4 : Outport  Port=5
  wires:
  sync/1 -> square_transposer/1(sync)
  square_transposer/1(sync_out) -> reorder/1(sync)
  reorder/1(sync_out) -> sync_out/1
  const/1 -> reorder/2(en)
  In1/1 -> square_transposer/2(In1)
  square_transposer/2(Out1) -> reorder/3(din0)
  reorder/3(dout0) -> Out1/1
  In2/1 -> square_transposer/3(In2)
  square_transposer/3(Out2) -> reorder/4(din1)
  reorder/4(dout1) -> Out2/1
  In3/1 -> square_transposer/4(In3)
  square_transposer/4(Out3) -> reorder/5(din2)
  reorder/5(dout2) -> Out3/1
  In4/1 -> square_transposer/5(In4)
  square_transposer/5(Out4) -> reorder/6(din3)
  reorder/6(dout3) -> Out4/1

== system casper_library/FFTs/fft_wideband_real ==
  sync : Inport  Port=1  LatchInput=off
  shift : Inport  Port=2  LatchInput=off
  in0 : Inport  Port=3  LatchInput=off
  in1 : Inport  Port=4  LatchInput=off
  in2 : Inport  Port=5  LatchInput=off
  in3 : Inport  Port=6  LatchInput=off
  fft_biplex_real_4x0 : Subsystem  AncestorBlock=casper_library/FFTs/fft_biplex_real_4x  mask(fft_biplex_real_4x){FFTSize=3, BitWidth=18, quantization=Truncate, overflow=Wrap, add_latency=2, mult_latency=3, bram_latency=2}
      mask prompts: FFTSize "Size of FFT: (2^? pnts)"; BitWidth "Bitwidth: (Max Efficiency at 18 bits)"; quantization "Quantization Behavior"; overflow "Overflow Behavior"; add_latency "Add Latency"; mult_latency "Mult Latency"; bram_latency "BRAM Latency"
      mask init: same as casper_library/FFTs/fft_biplex_real_4x
      settings: AttributesFormatString=FFTSize=3, BitWidth=18
      mask StyleString: edit,edit,popup(Truncate|Round  (unbiased: +/- Inf)|Round  (unbiased: Even Values)),popup(Wrap|Saturate|Error),edit,edit,edit
  fft_direct : Subsystem  AncestorBlock=casper_library/FFTs/fft_direct  mask(fft_direct){FFTSize=2, BitWidth=18, add_latency=2, mult_latency=3, bram_latency=2, quantization=Truncate, overflow=Wrap, MapTail=1, LargerFFTSize=5, StartStage=4}
      mask prompts: FFTSize "Size of FFT: (2^?)"; BitWidth "Bit Width"; add_latency "Add Latency"; mult_latency "Mult Latency"; bram_latency "BRAM Latency"; quantization "Quantization Behavior"; overflow "Overflow Behavior"; MapTail "Map Tail of Larger FFT"; LargerFFTSize "Size of Larger FFT (2^?):"; StartStage "Start Stage of Map Tail:"
      mask init: same as casper_library/FFTs/fft_direct
      settings: AttributesFormatString=FFTSize=2
      mask StyleString: edit,edit,edit,edit,edit,popup(Truncate|Round  (unbiased: +/- Inf)|Round  (unbiased: Even Values)),popup(Wrap|Saturate|Error),edit,edit,edit
  fft_unscrambler : Subsystem  AncestorBlock=casper_library/FFTs/fft_unscrambler  mask(fft_unscrambler){FFTSize=4, n_inputs=1, bram_latency=2}
      mask prompts: FFTSize "Size of FFT: (2^?)"; n_inputs "Number of Simultaneous Inputs: (2^?)"; bram_latency "BRAM Latency"
      mask init:
      | fft_unscrambler_init(gcb,...
      |     'FFTSize',FFTSize,... 
      |     'n_inputs', n_inputs,...
      |     'bram_latency', bram_latency);
      settings: AttributesFormatString=FFTSize=4, n_inputs=1
  slice : xbsIndex_r3/Slice  mode=Lower Bit Location + Width  nbits=2  bit1=0  base1=MSB of Input  bit0=3  base0=LSB of Input  boolean_output=off  explicit_period=off  period=1  dbl_ovrd=off
  sync_out : Outport
  out0 : Outport  Port=2
  out1 : Outport  Port=3
  wires:
  in0/1 -> fft_biplex_real_4x0/1(pol1)
  in1/1 -> fft_biplex_real_4x0/2(pol2)
  in2/1 -> fft_biplex_real_4x0/3(pol3)
  in3/1 -> fft_biplex_real_4x0/4(pol4)
  shift/1 -> fft_biplex_real_4x0/6(shift), slice/1
  sync/1 -> fft_biplex_real_4x0/5(sync)
  slice/1 -> fft_direct/2(shift)
  fft_biplex_real_4x0/6(sync_out) -> fft_direct/1(sync)
  fft_biplex_real_4x0/1(pol1_out) -> fft_direct/3(in0)
  fft_biplex_real_4x0/2(pol2_out) -> fft_direct/4(in1)
  fft_biplex_real_4x0/3(pol3_out) -> fft_direct/5(in2)
  fft_biplex_real_4x0/4(pol4_out) -> fft_direct/6(in3)
  fft_direct/1(sync_out) -> fft_unscrambler/1(sync)
  fft_unscrambler/1(sync_out) -> sync_out/1
  fft_direct/2(out0) -> fft_unscrambler/2(In1)
  fft_unscrambler/2(Out1) -> out0/1
  fft_direct/3(out1) -> fft_unscrambler/3(In2)
  fft_unscrambler/3(Out2) -> out1/1

== system casper_library/FFTs/map ==
  din : Inport  Port=1  LatchInput=off
  Concat : xbsIndex_r3/Concat  num_inputs=4  explicit_period=off  period=1  dbl_ovrd=off
  Uncram : casper_library/Misc/uncram  num_slice=4  slice_width=1  bin_pt=0  arith_type=0
      settings: AttributesFormatString=UFix_1_0
  expr0 : xbsIndex_r3/Expression  expression=(in03)|(in00&~in00)|(in01&~in01)|(in02&~in02)|(in03&~in03)  precision=Full  arith_type=Unsigned  n_bits=8  bin_pt=2  align_bp=on  latency=1  explicit_period=off  period=1  en=off  dbl_ovrd=off  show_param=off
      settings: xl_area=[0, 0, 0, 0, 0, 0, 0]
  expr1 : xbsIndex_r3/Expression  expression=(in02)|(in00&~in00)|(in01&~in01)|(in02&~in02)|(in03&~in03)  precision=Full  arith_type=Unsigned  n_bits=8  bin_pt=2  align_bp=on  latency=1  explicit_period=off  period=1  en=off  dbl_ovrd=off  show_param=off
      settings: xl_area=[0, 0, 0, 0, 0, 0, 0]
  expr2 : xbsIndex_r3/Expression  expression=(in01)|(in00&~in00)|(in01&~in01)|(in02&~in02)|(in03&~in03)  precision=Full  arith_type=Unsigned  n_bits=8  bin_pt=2  align_bp=on  latency=1  explicit_period=off  period=1  en=off  dbl_ovrd=off  show_param=off
      settings: xl_area=[0, 0, 0, 0, 0, 0, 0]
  expr3 : xbsIndex_r3/Expression  expression=(in00)|(in00&~in00)|(in01&~in01)|(in02&~in02)|(in03&~in03)  precision=Full  arith_type=Unsigned  n_bits=8  bin_pt=2  align_bp=on  latency=1  explicit_period=off  period=1  en=off  dbl_ovrd=off  show_param=off
      settings: xl_area=[0, 0, 0, 0, 0, 0, 0]
  dout : Outport
  wires:
  ? -> expr0/1, expr1/1, expr2/1, expr3/1
  ? -> expr0/2, expr1/2, expr2/2, expr3/2
  Uncram/2 -> expr0/3, expr1/3, expr2/3, expr3/3
  Uncram/1 -> expr0/4, expr1/4, expr2/4, expr3/4
  expr0/1 -> Concat/4
  expr1/1 -> Concat/3
  expr2/1 -> Concat/2
  expr3/1 -> Concat/1
  din/1 -> Uncram/1
  Concat/1 -> dout/1
